simulink library "controller"  (R2012b)
settings: Solver=ode45  StartTime=0.0  StopTime=10.0  RelTol=1e-3
values from neighbouring files (symbols this model uses):
  control =     [TruckBenchmark_Control.mat]
  road = scenario.road    [runSim.m]
libraries: simulink x1
settings Model: Creator=larer  LastModifiedBy=andth44

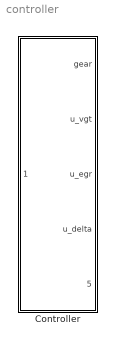
== system controller ==
  Controller : Subsystem

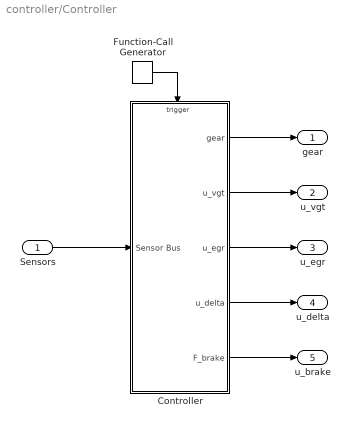
== system controller/Controller ==
  Sensors : Inport
  Controller : Subsystem  TreatAsAtomicUnit=on  SystemSampleTime=0.1
      settings: MinAlgLoopOccurrences=on  PropExecContextOutsideSubsystem=on
  Function-Call Generator : simulink/Ports & Subsystems/Function-Call Generator  sample_time=control.Ts  numberOfIterations=1
  gear : Outport
  u_vgt : Outport  Port=2
  u_egr : Outport  Port=3
  u_delta : Outport  Port=4
  u_brake : Outport  Port=5
  wires:
  Sensors/1 -> Controller/1(Sensor Bus)
  Controller/5(F_brake) -> u_brake/1
  Controller/3(u_egr) -> u_egr/1
  Function-Call Generator/1 -> Controller/Trigger
  Controller/4(u_delta) -> u_delta/1
  Controller/1(gear) -> gear/1
  Controller/2(u_vgt) -> u_vgt/1

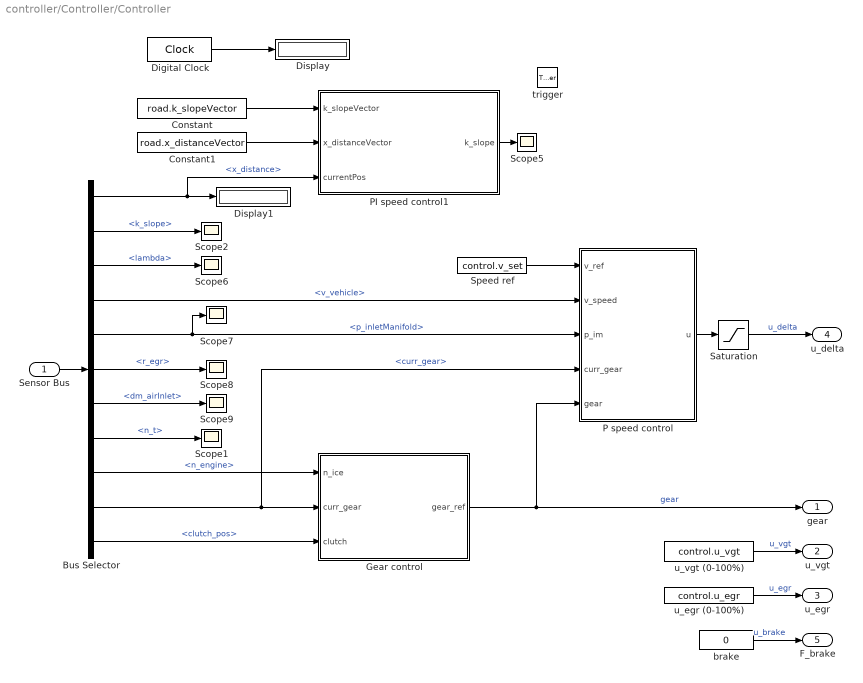
== system controller/Controller/Controller ==
  Sensor Bus : Inport
  trigger : TriggerPort  TriggerType=function-call  PortDimensions=1
  Bus Selector : BusSelector  OutputSignals=x_distance,k_slope,lambda,v_vehicle,p_inletManifold,r_egr,dm_airInlet,n_t,n_engine,curr_gear,clutch_pos
  Constant : Constant  Value=road.k_slopeVector
  Constant1 : Constant  Value=road.x_distanceVector
  Digital Clock : DigitalClock  SampleTime=-1
  Display : Display
  Display1 : Display
  Gear control : MATLAB Function  TreatAsAtomicUnit=on
      settings: PermitHierarchicalResolution=ParametersOnly
  P speed control : MATLAB Function  TreatAsAtomicUnit=on
      settings: PermitHierarchicalResolution=ParametersOnly
  PI speed control1 : MATLAB Function  TreatAsAtomicUnit=on
      settings: PermitHierarchicalResolution=ParametersOnly
  Saturation : Saturate  UpperLimit=300  LowerLimit=0
  Scope{1..2,5..9} (7 alike) : Scope
      Scope1 settings: YMin=-116.667  YMax=-105.555
      Scope2 settings: YMin=-116.667  YMax=-105.555  SaveName=ScopeData35
      Scope5 settings: YMin=-116.667  YMax=-105.555  SaveName=ScopeData47
      Scope6 settings: YMin=-116.667  YMax=-105.555  SaveName=ScopeData48
      Scope7 settings: YMin=-116.667  YMax=-105.555  SaveName=ScopeData49
      Scope8 settings: YMin=-116.667  YMax=-105.555  SaveName=ScopeData50
      Scope9 settings: YMin=-116.667  YMax=-105.555  SaveName=ScopeData51
  Speed ref : Constant  Value=control.v_set
  brake : Constant  Value=0
  u_egr (0-100%) : Constant  Value=control.u_egr
  u_vgt (0-100%) : Constant  Value=control.u_vgt
  gear : Outport  InitialOutput=0
  u_vgt : Outport  Port=2  InitialOutput=0
  u_egr : Outport  Port=3  InitialOutput=0
  u_delta : Outport  Port=4  InitialOutput=0
  F_brake : Outport  Port=5  InitialOutput=0
  wires:
  Bus Selector/11 -> Gear control/3(clutch)  "<clutch_pos>"
  Gear control/1(gear_ref) -> P speed control/5(gear), gear/1  "gear"
  Bus Selector/10 -> P speed control/4(curr_gear), Gear control/2(curr_gear)  "<curr_gear>"
  P speed control/1(u) -> Saturation/1
  Bus Selector/8 -> Scope1/1  "<n_t>"
  Bus Selector/4 -> P speed control/2(v_speed)  "<v_vehicle>"
  Bus Selector/9 -> Gear control/1(n_ice)  "<n_engine>"
  Bus Selector/7 -> Scope9/1  "<dm_airInlet>"
  Bus Selector/2 -> Scope2/1  "<k_slope>"
  Bus Selector/6 -> Scope8/1  "<r_egr>"
  Bus Selector/1 -> PI speed control1/3(currentPos), Display1/1  "<x_distance>"
  Bus Selector/3 -> Scope6/1  "<lambda>"
  Bus Selector/5 -> P speed control/3(p_im), Scope7/1  "<p_inletManifold>"
  Sensor Bus/1 -> Bus Selector/1
  PI speed control1/1(k_slope) -> Scope5/1
  Constant1/1 -> PI speed control1/2(x_distanceVector)
  Constant/1 -> PI speed control1/1(k_slopeVector)
  Digital Clock/1 -> Display/1
  brake/1 -> F_brake/1  "u_brake"
  u_egr (0-100%)/1 -> u_egr/1  "u_egr"
  u_vgt (0-100%)/1 -> u_vgt/1  "u_vgt"
  Saturation/1 -> u_delta/1  "u_delta"
  Speed ref/1 -> P speed control/1(v_ref)

== matlab function controller/Controller/Controller/P speed control ==
  data: v_ref input; v_speed input; u output; p_im input; curr_gear input; gear input
function u  = P(v_ref,v_speed,p_im,curr_gear,gear)
%#codegen


Kp      = 300;
v_err   = v_ref - v_speed;
u       = v_err * Kp;

% smoke limiter
K_smoke = 0.0012;
u_max=K_smoke*p_im;

% handle upshifts where the speed changes rapidly and the slowly sampled
% controller lags behind.
persistent last_gear second_last_gear

if isempty(last_gear)
  last_gear=4;
  second_last_gear=4;
end
if second_last_gear<curr_gear,
  u_max=u_max*.7;
end

second_last_gear=last_gear;
last_gear=curr_gear;
u=min(u,u_max);

== matlab function controller/Controller/Controller/PI speed control1 ==
  data: k_slopeVector input; k_slope output; x_distanceVector input; currentPos input
function k_slope = slope(k_slopeVector ,  x_distanceVector, currentPos)
%#codegen

% This function is not implemented.
k_slope      = 0;

== matlab function controller/Controller/Controller/Gear control ==
  data: n_ice input; gear_ref output; curr_gear input; clutch input
function gear_ref  = gearbox_control(n_ice, curr_gear, clutch)
%#codegen

% Define persistant variables
persistent curr_gear_ref

% initialize persistant variable
if isempty(curr_gear_ref)
    curr_gear_ref=4;
end

n_gearUpshift = 1250;
n_gearDoubleUpshift = 1800;
n_gearDownshift = 900;
gearMax   = 14;
gearMin   = 4;

if curr_gear_ref~=curr_gear || clutch~=1; %Gear in progress - keep current gear reference
    gear_ref = curr_gear_ref;     
elseif n_ice > n_gearUpshift && curr_gear < gearMax %Shift upp  
    if n_ice > n_gearDoubleUpshift && curr_gear < gearMax-1 %Shift up two gears
        gear_ref = curr_gear + 2;
    else % Shift up one gear
        gear_ref = curr_gear + 1;
    end 
elseif n_ice < n_gearDownshift && curr_gear > gearMin %Shift down
    gear_ref = curr_gear - 1;
else %No shift - keep current gear
    gear_ref = curr_gear;
end

gear_ref = min(max(gear_ref,gearMin),gearMax); %Should not be necissairy

curr_gear_ref=gear_ref;
